simulink library "INT_PTOSwt_DD"  (R2016b)
settings: Solver=VariableStepAuto  StartTime=0.0  StopTime=10.0  RelTol=1e-3
settings Model: Creator=liutao  LastModifiedBy=liutao

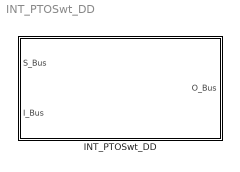
== system INT_PTOSwt_DD ==
  INT_PTOSwt_DD : Subsystem

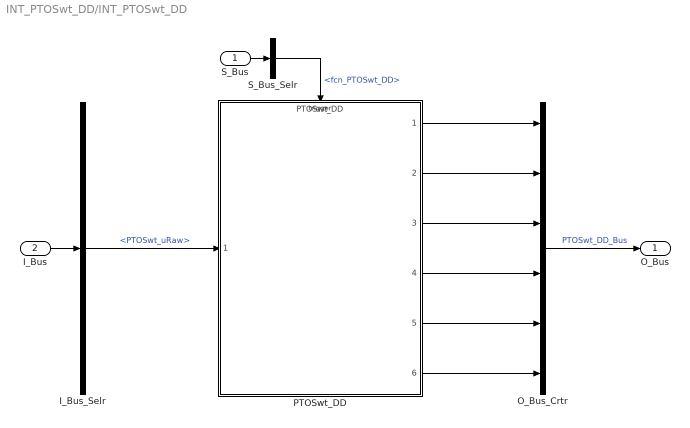
== system INT_PTOSwt_DD/INT_PTOSwt_DD ==
  S_Bus : Inport
  I_Bus : Inport  Port=2
  I_Bus_Selr : BusSelector  OutputSignals=PTOSwt_uRaw
  O_Bus_Crtr : BusCreator  Inputs=6
  PTOSwt_DD : ModelReference  ModelNameDialog=PTOSwt_DD  SimulationMode=Normal  ModelReferenceVersion=1.19  TriggerPortName=function  TriggerPortTriggerType=function-call  TriggerPortStatesWhenEnabling=held
  S_Bus_Selr : BusSelector  OutputSignals=fcn_PTOSwt_DD
  O_Bus : Outport
  wires:
  S_Bus_Selr/1 -> PTOSwt_DD/Trigger  "<fcn_PTOSwt_DD>"
  S_Bus/1 -> S_Bus_Selr/1
  I_Bus/1 -> I_Bus_Selr/1
  I_Bus_Selr/1 -> PTOSwt_DD/1  "<PTOSwt_uRaw>"
  O_Bus_Crtr/1 -> O_Bus/1  "PTOSwt_DD_Bus"
  PTOSwt_DD/1 -> O_Bus_Crtr/1
  PTOSwt_DD/2 -> O_Bus_Crtr/2
  PTOSwt_DD/3 -> O_Bus_Crtr/3
  PTOSwt_DD/4 -> O_Bus_Crtr/4
  PTOSwt_DD/5 -> O_Bus_Crtr/5
  PTOSwt_DD/6 -> O_Bus_Crtr/6
